simulink model "SRT2ARL"  (R2024b)
settings: Solver=FixedStepAuto  StartTime=0.0  StopTime=3  FixedStep=0.01  RelTol=1e-3
values from neighbouring files (symbols this model uses):
  theta0 = 0    [msdResetFcn.m]
  thetad0 = 0    [msdResetFcn.m]
  x0 = 0.5    [msdResetFcn.m]
  y0 = 0    [msdResetFcn.m]
libraries: simulink x1, rllib x1
settings Model: Creator=Robin  LastModifiedBy=Robin
settings DebuggingCC: UniqueDataStoreMsg=error

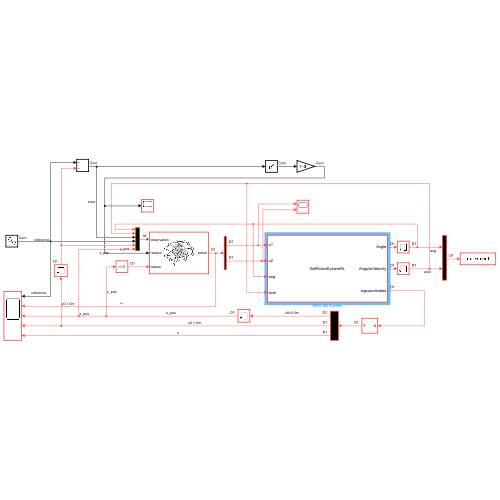
[thumbnail: Simulink's stored preview of the top-level diagram]
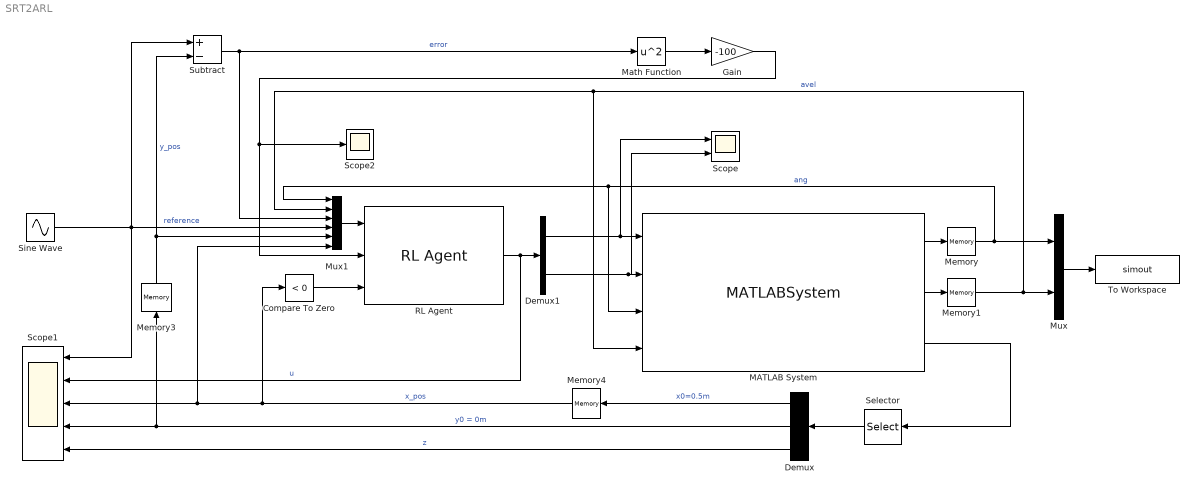
== system SRT2ARL ==
  Compare To Zero : simulink/Logic and Bit Operations/Compare To Zero  relop=<  OutDataTypeStr=boolean
  Demux : Demux  Outputs=3
  Demux1 : Demux  Outputs=2
  Gain : Gain  Gain=-100
  MATLAB System : MATLABSystem  System=SoftRobotSystemRL  SimulateUsing=Interpreted execution
      mask Type: SoftRobotSystemRL
      mask Display:
      | disp('SoftRobotSystemRL');
      | port_label('input',1,'u1');
      | port_label('input',2,'u2');
      | port_label('input',3,'ang');
      | port_label('input',4,'avel');
      | port_label('output',1,'Angle');
      | port_label('output',2,'AngularVelocity');
      | port_label('output',3,'sigcoordinates');
  Math Function : Math  Operator=square
  Memory : Memory  InitialCondition=theta0
  Memory1 : Memory  InitialCondition=thetad0
  Memory3 : Memory  InitialCondition=y0
  Memory4 : Memory  InitialCondition=x0
  Mux : Mux  Inputs=2
  Mux1 : Mux  Inputs=6
  RL Agent : rllib/RL Agent  Agent=agent  ExternalActionAsInput=off  ProvideLastAction=off  ProvideCumRwd=off  TreatAsDirectFeedthrough=on  UseStrictObservationDataTypes=off
  Scope : Scope  NumInputPorts=2
  Scope1 : Scope  NumInputPorts=5
  Scope2 : Scope
  Selector : Selector  InputPortWidth=24  IndexOptions=Index vector (dialog)  Indices=[22 23 24]  OutputSizes=1
  Sine Wave : Sin  Amplitude=0.3  SampleTime=0
  Subtract : Sum  Inputs=+-
  To Workspace : ToWorkspace  VariableName=simout  SampleTime=-1
  wires:
  Sine Wave/1 -> Subtract/1, Scope1/1, Mux1/4  "reference"
  MATLAB System/1 -> Memory/1
  MATLAB System/2 -> Memory1/1
  MATLAB System/3 -> Selector/1
  Memory/1 -> Mux/1, MATLAB System/3, Mux1/1  "ang"
  Memory1/1 -> MATLAB System/4, Mux1/2, Mux/2  "avel"
  Mux/1 -> To Workspace/1
  Demux/1 -> Memory4/1  "x0=0.5m"
  Demux/2 -> Memory3/1, Scope1/4  "y0 = 0m"
  Demux/3 -> Scope1/5  "z"
  Selector/1 -> Demux/1
  Memory3/1 -> Subtract/2, Mux1/5  "y_pos"
  Mux1/1 -> RL Agent/1
  Subtract/1 -> Mux1/3, Math Function/1  "error"
  RL Agent/1 -> Scope1/2, Demux1/1  "u"
  Demux1/1 -> Scope/1, MATLAB System/1
  Demux1/2 -> Scope/2, MATLAB System/2
  Math Function/1 -> Gain/1
  Gain/1 -> RL Agent/2, Scope2/1
  Memory4/1 -> Compare To Zero/1, Mux1/6, Scope1/3  "x_pos"
  Compare To Zero/1 -> RL Agent/3
